simulink model "main_sim_noadapt"  (Simulink 7.2)
settings: Solver=ode2  SolverMode=SingleTasking  StartTime=0.0  StopTime=tsim_max  FixedStep=dtsim  RelTol=1e-3
StopFcn:
  | %mkplt
values from neighbouring files (symbols this model uses):
  vel = 128    [do_command_tracking.m]
undefined symbols (not defined in the file or in its folder): accel_cmd, aero_surf_qbar_off, aero_surf_qbar_on, assertion_time, att_cmd_select, att_trim_IC, att_type, att_type_numbers, bb_ellipsoid, bb_params, chi_trim_IC, command_time, compute_all_rate_cols, compute_all_vel_cols, constants, cosA, da_trim_IC, dc_L2W_IC, de_trim_IC, DiscIntNeverNeededParam, dr_trim_IC, dtsim, E_rwy, E_trim_IC, Ed_cmd, Ed_trim_IC, eow_boundary, flag_exsig, full_surf_llim, full_surf_ulim, gain_set, gain_var_struct, gam_cmd_descent, gam_cmd_preflare, gamdot_cmd_descent, gamdot_cmd_flare, gamdot_cmd_preflare, gamma_trim_IC, h_trim_IC, hd_cmd, hd_trim_IC, ideal_vel_Kb, in_exsig_vecin, in_exsig_vecout, in_t_exsig, MACH, MACH_att_fb, MACH_att_int_IC, MACH_att_Kb, MACH_att_Kc, MACH_att_Ki, MACH_gain_mat, MACH_mass_IC, MACH_pos_IC, MACH_pos_int_IC, MACH_pos_Kb, MACH_pos_Kc, MACH_pos_Ki, MACH_pqr_Bmat_IC, MACH_pqr_IC ... (+62)
libraries: simulink x36, utility_lib x34, mach_lib x24, model_lib x13, simulink_need_slupdate x8, models x8
(part 2 of 7)

== system main_sim_noadapt/vehicle_model/target/seeker model ==
  output_bus : Inport  OutDataType=sfix(16)  OutScaling=2^0
  Bus Selector : BusSelector  OutputSignals=x,xdot
  Bus Selector1 : BusSelector  OutputSignals=LOS_rate,aux_info.azimuth,aux_info.elevation,aux_info.Rground,aux_info.Rslant
  Constant2 : Constant  Value=target_vel_IC  OutDataType=sfix(16)  OutScaling=2^0
  NEh : Selector  InputPortWidth=MACH.num_x  IndexOptions=Index vector (dialog)  Indices=MACH.NEh_idx  OutputSizes=1
  NEh_dot : Selector  InputPortWidth=MACH.num_x  IndexOptions=Index vector (dialog)  Indices=MACH.NEh_idx  OutputSizes=1
  seeker model : Subsystem
  seeker scope : Scope  NumInputPorts=5
      settings: YMin=-1.75~-3.5~-1.75~0~0  YMax=0.25~0.5~0~450000~550000
  target position integrator : Integrator  InitialCondition=target_pos_IC
  seeker : Outport  OutDataType=sfix(16)  OutScaling=2^0
  wires:
  Constant2/1 -> target position integrator/1, seeker model/2(NEh_d_target)
  target position integrator/1 -> seeker model/1(NEh_target)
  NEh/1 -> seeker model/3(NEh)
  NEh_dot/1 -> seeker model/4(NEh_d)
  seeker model/1(seeker) -> seeker/1, Bus Selector1/1
  output_bus/1 -> Bus Selector/1
  Bus Selector/1 -> NEh/1  "<x>"
  Bus Selector/2 -> NEh_dot/1  "<xdot>"
  Bus Selector1/2 -> seeker scope/2  "<azimuth>"
  Bus Selector1/3 -> seeker scope/3  "<elevation>"
  Bus Selector1/4 -> seeker scope/4  "<Rground>"
  Bus Selector1/5 -> seeker scope/5  "<Rslant>"
  Bus Selector1/1 -> seeker scope/1  "<LOS_rate>"

== system main_sim_noadapt/claw_main/att_loops/P+I+AW+TRIM Control ==
  cv : Inport  OutDataType=sfix(16)  OutScaling=2^0
  cv cmd : Inport  Port=2  OutDataType=sfix(16)  OutScaling=2^0
  cvd ff : Inport  Port=3  OutDataType=sfix(16)  OutScaling=2^0
  cvdot extra : Inport  Port=4  OutDataType=sfix(16)  OutScaling=2^0
  trim : Inport  Port=5  OutDataType=sfix(16)  OutScaling=2^0
  reset : Inport  Port=6  OutDataType=sfix(16)  OutScaling=2^0
  x0 : Inport  Port=7  OutDataType=sfix(16)  OutScaling=2^0
  Dot Product2 : simulink/Math Operations/Dot Product  InputSameDT=on  OutDataType=sfix(16)  OutScaling=2^-10  DoSatur=off
  P+I+AW+TRIM Control : mach_lib/P+I+AW+TRIM Control  SystemSampleTime=-1
  Product2 : Product  OutDataType=sfix(16)  OutScaling=2^0  SaturateOnIntegerOverflow=on  InputSameDT=on  OutDataTypeStr=Inherit: Same as first input
  Sum : Sum  Inputs=-+|  OutDataType=sfix(16)  OutScaling=2^0  SaturateOnIntegerOverflow=on
  Unit Delay1 : UnitDelay  SampleTime=-1
  fe : Gain  Gain=MACH.att_fe  ParameterDataType=sfix(16)  ParameterScaling=2^0  OutDataType=sfix(16)  OutScaling=2^0  SaturateOnIntegerOverflow=on  OutDataTypeStr=Inherit: Same as input  ParamDataTypeStr=Inherit: Same as input
  cvdot des : Outport  OutDataType=sfix(16)  OutScaling=2^0
  int state : Outport  Port=2  OutDataType=sfix(16)  OutScaling=2^0
  wires:
  cvd ff/1 -> P+I+AW+TRIM Control/3
  cvdot extra/1 -> P+I+AW+TRIM Control/4
  Sum/1 -> P+I+AW+TRIM Control/5
  reset/1 -> P+I+AW+TRIM Control/6
  x0/1 -> P+I+AW+TRIM Control/7
  fe/1 -> Sum/1
  trim/1 -> Sum/2
  Product2/1 -> fe/1
  Unit Delay1/1 -> Dot Product2/2
  Dot Product2/1 -> Product2/2
  P+I+AW+TRIM Control/2 -> int state/1
  P+I+AW+TRIM Control/1 -> Unit Delay1/1, cvdot des/1
  cv cmd/1 -> P+I+AW+TRIM Control/2
  cv/1 -> Product2/1, Dot Product2/1, P+I+AW+TRIM Control/1

== system main_sim_noadapt/claw_main/att_loops/compute trim ==
  inner cmd : Inport  OutDataType=sfix(16)  OutScaling=2^0
  Bmat : Inport  Port=2  OutDataType=sfix(16)  OutScaling=2^0
  cmd : Inport  Port=3  OutDataType=sfix(16)  OutScaling=2^0
  Product : Product  Multiplication=Matrix(*)  OutDataType=sfix(16)  OutScaling=2^0  SaturateOnIntegerOverflow=on  OutDataTypeStr=Inherit: Same as first input
  Sum1 : Sum  Inputs=|+-  OutDataType=sfix(16)  OutScaling=2^0  SaturateOnIntegerOverflow=on
  trim : Outport  OutDataType=sfix(16)  OutScaling=2^0
  wires:
  Product/1 -> trim/1
  Bmat/1 -> Product/1
  Sum1/1 -> Product/2
  inner cmd/1 -> Sum1/1
  cmd/1 -> Sum1/2

== system main_sim_noadapt/claw_main/att_loops/dyn inv ==
  limit_pqr_cmd : Inport  OutDataType=sfix(16)  OutScaling=2^0
  uvw : Inport  Port=2  OutDataType=sfix(16)  OutScaling=2^0
  e nom : Inport  Port=3  OutDataType=sfix(16)  OutScaling=2^0
  e dot des : Inport  Port=4  OutDataType=sfix(16)  OutScaling=2^0
  Dot Product : simulink/Math Operations/Dot Product  InputSameDT=on  OutDataType=sfix(16)  OutScaling=2^-10  DoSatur=off
  Gain4 : Gain  Gain=0.5  ParameterDataType=sfix(16)  ParameterScaling=2^0  OutDataType=sfix(16)  OutScaling=2^0
  Limit rate cmd : Subsystem
  Product4 : Product  OutDataType=sfix(16)  OutScaling=2^0  SaturateOnIntegerOverflow=on  InputSameDT=on  OutDataTypeStr=Inherit: Same as first input
  Product5 : Product  Inputs=**  Multiplication=Matrix(*)  OutDataType=sfix(16)  OutScaling=2^0  SaturateOnIntegerOverflow=on  InputSameDT=on  OutDataTypeStr=Inherit: Same as first input
  Sum4 : Sum  Inputs=++-  OutDataType=sfix(16)  OutScaling=2^0  SaturateOnIntegerOverflow=on  InputSameDT=on  OutDataTypeStr=Inherit: Same as first input
  getedinv : utility_lib/getedinv  SystemSampleTime=-1
  Bmat : Outport  OutDataType=sfix(16)  OutScaling=2^0
  pqr : Outport  Port=2  OutDataType=sfix(16)  OutScaling=2^0
  cvdex : Outport  Port=3  OutDataType=sfix(16)  OutScaling=2^0
  wires:
  Limit rate cmd/1(pqr_limited) -> pqr/1, Product5/2
  Sum4/1 -> cvdex/1
  Product4/1 -> Sum4/2
  Product5/1 -> Sum4/1
  e dot des/1 -> Dot Product/2, Sum4/3, getedinv/1
  e nom/1 -> Product4/1, Dot Product/1, getedinv/2
  Dot Product/1 -> Product4/2
  getedinv/2 -> Gain4/1
  uvw/1 -> Limit rate cmd/2(uvw)
  getedinv/1 -> Limit rate cmd/3(pqr)
  limit_pqr_cmd/1 -> Limit rate cmd/1(limit_pqr_cmd)
  Gain4/1 -> Product5/1, Bmat/1

== system main_sim_noadapt/claw_main/att_loops/low pass filter ==
  e_cmd : Inport  OutDataType=sfix(16)  OutScaling=2^0
  signal_bus : Inport  Port=2  OutDataType=sfix(16)  OutScaling=2^0
  att_ff : Inport  Port=3  OutDataType=sfix(16)  OutScaling=2^0
  Bus Selector4 : BusSelector  OutputSignals=control_params.att_desdyn.kf,control_params.att_desdyn.kb
  Compare To Zero : simulink/Logic and Bit Operations/Compare To Zero  SystemSampleTime=-1  relop===  LogicOutDataTypeMode=boolean  ZeroCross=off
  Constant : Constant  Value=MACH_att_fb  OutDataType=sfix(16)  OutScaling=2^0
  Discrete-Time Integrator : DiscreteIntegrator  ExternalReset=sampled level  InitialConditionSource=external  SampleTime=-1  OutDataType=sfix(16)  OutScaling=2^0  ICPrevOutput=DiscIntNeverNeededParam  ICPrevScaledInput=DiscIntNeverNeededParam
  Product : Product  Inputs=3  OutDataType=sfix(16)  OutScaling=2^0  RndMeth=Zero
  Product1 : Product  OutDataType=sfix(16)  OutScaling=2^0  RndMeth=Zero
  Product2 : Product  OutDataType=sfix(16)  OutScaling=2^0  RndMeth=Zero
  Sum : Sum  Inputs=|+-  OutDataType=sfix(16)  OutScaling=2^0
  Sum1 : Sum  Inputs=++|  OutDataType=sfix(16)  OutScaling=2^0
  cv cmd : Outport  OutDataType=sfix(16)  OutScaling=2^0
  cvd ff : Outport  Port=2  OutDataType=sfix(16)  OutScaling=2^0
  wires:
  Product/1 -> Sum1/2
  e_cmd/1 -> Sum/1, Discrete-Time Integrator/3
  Sum/1 -> Product/3
  Sum1/1 -> Discrete-Time Integrator/1, cvd ff/1
  Discrete-Time Integrator/1 -> Sum/2, cv cmd/1
  signal_bus/1 -> Bus Selector4/1
  att_ff/1 -> Product1/1
  Product1/1 -> Sum1/1
  Compare To Zero/1 -> Discrete-Time Integrator/2
  Bus Selector4/2 -> Product/2  "<kb>"
  Product2/1 -> Product/1, Compare To Zero/1
  Bus Selector4/1 -> Product2/2, Product1/2  "<kf>"
  Constant/1 -> Product2/1

== system main_sim_noadapt/claw_main/att_loops/select att cmd ==
  e_current : Inport  OutDataType=sfix(16)  OutScaling=2^0
  throt_current : Inport  Port=2  OutDataType=sfix(16)  OutScaling=2^0
  outer cmd : Inport  Port=3  OutDataType=sfix(16)  OutScaling=2^0
  signal_bus : Inport  Port=4  OutDataType=sfix(16)  OutScaling=2^0
  Bus Selector1 : BusSelector  OutputSignals=cmd_bus.select_cmd.att
  Compare To Zero : simulink/Logic and Bit Operations/Compare To Zero  SystemSampleTime=-1  relop===  LogicOutDataTypeMode=boolean  ZeroCross=off
  Demux : Demux  Outputs=[ 4 1 ]
  Demux1 : Demux  Outputs=[ 3 MACH.num_u_throt ]
  Demux2 : Demux  Outputs=[ 1 3 ]
  Mux1 : Mux  Inputs=2
  Switch : Switch  Threshold=0.5
  Unit Delay2 : UnitDelay  X0=MACH_throttle_IC  SampleTime=-1
  att2e_ref : utility_lib/att2e_ref  SystemSampleTime=-1
  e2att : utility_lib/e2att  SystemSampleTime=-1
  get direct cmd : Subsystem
  switch att cmd : MultiPortSwitch  zeroidx=on  SaturateOnIntegerOverflow=on
  switch throt cmd : MultiPortSwitch  zeroidx=on  SaturateOnIntegerOverflow=on
  e_cmd : Outport  OutDataType=sfix(16)  OutScaling=2^0
  throt_cmd : Outport  Port=2  OutDataType=sfix(16)  OutScaling=2^0
  cmd : Outport  Port=3  OutDataType=sfix(16)  OutScaling=2^0
  wires:
  switch att cmd/1 -> att2e_ref/1, Mux1/1
  Bus Selector1/1 -> Demux/1  "<att>"
  get direct cmd/2(throt) -> switch throt cmd/3
  throt_current/1 -> Unit Delay2/1
  Demux/2 -> switch throt cmd/1
  outer cmd/1 -> Demux1/1
  Demux1/2 -> switch throt cmd/4
  switch throt cmd/1 -> throt_cmd/1, Mux1/2
  signal_bus/1 -> get direct cmd/1(signal_bus), Bus Selector1/1
  Demux/1 -> Demux2/1
  e_current/1 -> e2att/1, Switch/1, att2e_ref/2
  Unit Delay2/1 -> switch throt cmd/2
  get direct cmd/1(att) -> switch att cmd/3
  e2att/1 -> switch att cmd/2
  Demux1/1 -> switch att cmd/4
  att2e_ref/1 -> Switch/3
  Switch/1 -> e_cmd/1
  Demux2/1 -> Compare To Zero/1
  Demux2/2 -> switch att cmd/1
  Compare To Zero/1 -> Switch/2
  Mux1/1 -> cmd/1

== system main_sim_noadapt/claw_main/grab ExportedGlobal/grab cv variables ==
  In1 : Inport  OutDataType=sfix(16)  OutScaling=2^0
  Bus Selector6 : BusSelector  OutputSignals=rate.cv,att.cv,vel.cv,pos.cv
  Demux1 : Demux  Outputs=3
  Demux2 : Demux
  Demux3 : Demux  Outputs=3
  Demux4 : Demux  Outputs=3
  Mux : Mux  Inputs=13
  Subsystem : Subsystem  TreatAsAtomicUnit=on
      settings: RTWSystemCode=Inline
  Out1 : Outport  OutDataType=sfix(16)  OutScaling=2^0
  wires:
  Subsystem/1(Out1) -> Mux/1  "CLAW_p_cv"
  Subsystem/2(Out2) -> Mux/2  "CLAW_q_cv"
  Subsystem/3(Out3) -> Mux/3  "CLAW_r_cv"
  Subsystem/4(Out4) -> Mux/4  "CLAW_e0_cv"
  Subsystem/5(Out5) -> Mux/5  "CLAW_e1_cv"
  Subsystem/6(Out6) -> Mux/6  "CLAW_e2_cv"
  Subsystem/8(Out8) -> Mux/8  "CLAW_Ndot_cv"
  Subsystem/9(Out9) -> Mux/9  "CLAW_Edot_cv"
  Subsystem/10(Out10) -> Mux/10  "CLAW_hdot_cv"
  Subsystem/11(Out11) -> Mux/11  "CLAW_N_cv"
  Subsystem/12(Out12) -> Mux/12  "CLAW_E_cv"
  Subsystem/13(Out13) -> Mux/13  "CLAW_h_cv"
  Subsystem/7(Out7) -> Mux/7  "CLAW_e3_cv"
  In1/1 -> Bus Selector6/1
  Mux/1 -> Out1/1
  Demux1/1 -> Subsystem/1(In1)
  Demux1/2 -> Subsystem/2(In2)
  Demux1/3 -> Subsystem/3(In3)
  Demux2/1 -> Subsystem/4(In4)
  Demux2/2 -> Subsystem/5(In5)
  Demux2/3 -> Subsystem/6(In6)
  Demux2/4 -> Subsystem/7(In7)
  Demux3/1 -> Subsystem/8(In8)
  Demux3/2 -> Subsystem/9(In9)
  Demux3/3 -> Subsystem/10(In10)
  Demux4/1 -> Subsystem/11(In11)
  Demux4/2 -> Subsystem/12(In12)
  Demux4/3 -> Subsystem/13(In13)
  Bus Selector6/1 -> Demux1/1  "<cv>"
  Bus Selector6/2 -> Demux2/1  "<cv>"
  Bus Selector6/3 -> Demux3/1  "<cv>"
  Bus Selector6/4 -> Demux4/1  "<cv>"

== system main_sim_noadapt/claw_main/grab ExportedGlobal/grab cvcmd variables ==
  In1 : Inport  OutDataType=sfix(16)  OutScaling=2^0
  Bus Selector5 : BusSelector  OutputSignals=rate.cvc,att.cvc,vel.cvc,pos.cvc
  Demux1 : Demux  Outputs=3
  Demux2 : Demux
  Demux3 : Demux  Outputs=3
  Demux4 : Demux  Outputs=3
  Mux : Mux  Inputs=13
  Subsystem : Subsystem  TreatAsAtomicUnit=on
      settings: RTWSystemCode=Inline
  Out1 : Outport  OutDataType=sfix(16)  OutScaling=2^0
  wires:
  Subsystem/1(Out1) -> Mux/1  "CLAW_p_cvcmd"
  Subsystem/2(Out2) -> Mux/2  "CLAW_q_cvcmd"
  Subsystem/3(Out3) -> Mux/3  "CLAW_r_cvcmd"
  Subsystem/4(Out4) -> Mux/4  "CLAW_e0_cvcmd"
  Subsystem/5(Out5) -> Mux/5  "CLAW_e1_cvcmd"
  Subsystem/6(Out6) -> Mux/6  "CLAW_e2_cvcmd"
  Subsystem/8(Out8) -> Mux/8  "CLAW_Ndot_cvcmd"
  Subsystem/9(Out9) -> Mux/9  "CLAW_Edot_cvcmd"
  Subsystem/10(Out10) -> Mux/10  "CLAW_hdot_cvcmd"
  Subsystem/11(Out11) -> Mux/11  "CLAW_N_cvcmd"
  Subsystem/12(Out12) -> Mux/12  "CLAW_E_cvcmd"
  Subsystem/13(Out13) -> Mux/13  "CLAW_h_cvcmd"
  Subsystem/7(Out7) -> Mux/7  "CLAW_e3_cvcmd"
  In1/1 -> Bus Selector5/1
  Mux/1 -> Out1/1
  Demux1/1 -> Subsystem/1(In1)
  Demux1/2 -> Subsystem/2(In2)
  Demux1/3 -> Subsystem/3(In3)
  Demux2/1 -> Subsystem/4(In4)
  Demux2/2 -> Subsystem/5(In5)
  Demux2/3 -> Subsystem/6(In6)
  Demux2/4 -> Subsystem/7(In7)
  Demux3/1 -> Subsystem/8(In8)
  Demux3/2 -> Subsystem/9(In9)
  Demux3/3 -> Subsystem/10(In10)
  Demux4/1 -> Subsystem/11(In11)
  Demux4/2 -> Subsystem/12(In12)
  Demux4/3 -> Subsystem/13(In13)
  Bus Selector5/4 -> Demux4/1  "<cvc>"
  Bus Selector5/2 -> Demux2/1  "<cvc>"
  Bus Selector5/1 -> Demux1/1  "<cvc>"
  Bus Selector5/3 -> Demux3/1  "<cvc>"

== system main_sim_noadapt/claw_main/grab ExportedGlobal/grab cvdex variables ==
  In1 : Inport  OutDataType=sfix(16)  OutScaling=2^0
  Bus Selector3 : BusSelector  OutputSignals=rate.cvdex,att.cvdex,vel.cvdex,pos.cvdex
  Demux1 : Demux  Outputs=3
  Demux2 : Demux
  Demux3 : Demux  Outputs=3
  Demux4 : Demux  Outputs=3
  Mux : Mux  Inputs=13
  Subsystem : Subsystem  TreatAsAtomicUnit=on
      settings: RTWSystemCode=Inline
  Out1 : Outport  OutDataType=sfix(16)  OutScaling=2^0
  wires:
  Subsystem/1(Out1) -> Mux/1  "CLAW_p_cvdex"
  Subsystem/2(Out2) -> Mux/2  "CLAW_q_cvdex"
  Subsystem/3(Out3) -> Mux/3  "CLAW_r_cvdex"
  Subsystem/4(Out4) -> Mux/4  "CLAW_e0_cvdex"
  Subsystem/5(Out5) -> Mux/5  "CLAW_e1_cvdex"
  Subsystem/6(Out6) -> Mux/6  "CLAW_e2_cvdex"
  Subsystem/8(Out8) -> Mux/8  "CLAW_Ndot_cvdex"
  Subsystem/9(Out9) -> Mux/9  "CLAW_Edot_cvdex"
  Subsystem/10(Out10) -> Mux/10  "CLAW_hdot_cvdex"
  Subsystem/11(Out11) -> Mux/11  "CLAW_N_cvdex"
  Subsystem/12(Out12) -> Mux/12  "CLAW_E_cvdex"
  Subsystem/13(Out13) -> Mux/13  "CLAW_h_cvdex"
  Subsystem/7(Out7) -> Mux/7  "CLAW_e3_cvdex"
  Demux1/1 -> Subsystem/1(In1)
  Demux1/2 -> Subsystem/2(In2)
  Demux1/3 -> Subsystem/3(In3)
  Demux2/1 -> Subsystem/4(In4)
  Demux2/2 -> Subsystem/5(In5)
  Demux2/3 -> Subsystem/6(In6)
  Demux2/4 -> Subsystem/7(In7)
  Demux3/1 -> Subsystem/8(In8)
  Demux3/2 -> Subsystem/9(In9)
  Demux3/3 -> Subsystem/10(In10)
  Demux4/1 -> Subsystem/11(In11)
  Demux4/2 -> Subsystem/12(In12)
  Demux4/3 -> Subsystem/13(In13)
  Mux/1 -> Out1/1
  In1/1 -> Bus Selector3/1
  Bus Selector3/4 -> Demux4/1  "<cvdex>"
  Bus Selector3/3 -> Demux3/1  "<cvdex>"
  Bus Selector3/2 -> Demux2/1  "<cvdex>"
  Bus Selector3/1 -> Demux1/1  "<cvdex>"

== system main_sim_noadapt/claw_main/grab ExportedGlobal/grab integrator variables ==
  In1 : Inport  OutDataType=sfix(16)  OutScaling=2^0
  Bus Selector4 : BusSelector  OutputSignals=rate.integ,att.integ,vel.integ,pos.integ
  Demux1 : Demux  Outputs=3
  Demux2 : Demux
  Demux3 : Demux  Outputs=3
  Demux4 : Demux  Outputs=3
  Mux : Mux  Inputs=13
  Subsystem : Subsystem  TreatAsAtomicUnit=on
      settings: RTWSystemCode=Inline
  Out1 : Outport  OutDataType=sfix(16)  OutScaling=2^0
  wires:
  Subsystem/1(Out1) -> Mux/1  "CLAW_p_int"
  Subsystem/2(Out2) -> Mux/2  "CLAW_q_int"
  Subsystem/3(Out3) -> Mux/3  "CLAW_r_int"
  Subsystem/4(Out4) -> Mux/4  "CLAW_e0_int"
  Subsystem/5(Out5) -> Mux/5  "CLAW_e1_int"
  Subsystem/6(Out6) -> Mux/6  "CLAW_e2_int"
  Subsystem/8(Out8) -> Mux/8  "CLAW_Ndot_int"
  Subsystem/9(Out9) -> Mux/9  "CLAW_Edot_int"
  Subsystem/10(Out10) -> Mux/10  "CLAW_hdot_int"
  Subsystem/11(Out11) -> Mux/11  "CLAW_N_int"
  Subsystem/12(Out12) -> Mux/12  "CLAW_E_int"
  Subsystem/13(Out13) -> Mux/13  "CLAW_h_int"
  Subsystem/7(Out7) -> Mux/7  "CLAW_e3_int"
  Mux/1 -> Out1/1
  Demux1/1 -> Subsystem/1(In1)
  Demux1/2 -> Subsystem/2(In2)
  Demux1/3 -> Subsystem/3(In3)
  Demux2/1 -> Subsystem/4(In4)
  Demux2/2 -> Subsystem/5(In5)
  Demux2/3 -> Subsystem/6(In6)
  Demux2/4 -> Subsystem/7(In7)
  Demux3/1 -> Subsystem/8(In8)
  Demux3/2 -> Subsystem/9(In9)
  Demux3/3 -> Subsystem/10(In10)
  Demux4/1 -> Subsystem/11(In11)
  Demux4/2 -> Subsystem/12(In12)
  Demux4/3 -> Subsystem/13(In13)
  In1/1 -> Bus Selector4/1
  Bus Selector4/4 -> Demux4/1  "<integ>"
  Bus Selector4/3 -> Demux3/1  "<integ>"
  Bus Selector4/2 -> Demux2/1  "<integ>"
  Bus Selector4/1 -> Demux1/1  "<integ>"

== system main_sim_noadapt/claw_main/grab ExportedGlobal/grab w_est variables ==
  In1 : Inport  OutDataType=sfix(16)  OutScaling=2^0
  Bus Selector12 : BusSelector  OutputSignals=w_est_debug.w_est
  Demux1 : Demux  Outputs=3
  Mux : Mux  Inputs=3
  Subsystem : Subsystem  TreatAsAtomicUnit=on
      settings: RTWSystemCode=Inline
  Out1 : Outport  OutDataType=sfix(16)  OutScaling=2^0
  wires:
  Subsystem/1(Out1) -> Mux/1  "CLAW_Nd_wind"
  Subsystem/2(Out2) -> Mux/2  "CLAW_Ed_wind"
  Subsystem/3(Out3) -> Mux/3  "CLAW_Dd_wind"
  Demux1/1 -> Subsystem/1(In1)
  Demux1/2 -> Subsystem/2(In2)
  Demux1/3 -> Subsystem/3(In3)
  Mux/1 -> Out1/1
  Bus Selector12/1 -> Demux1/1  "<w_est>"
  In1/1 -> Bus Selector12/1

== system main_sim_noadapt/claw_main/input processing/mode dependent stick processing ==
  command : Inport  OutDataType=sfix(16)  OutScaling=2^0
  signal_bus : Inport  Port=2  OutDataType=sfix(16)  OutScaling=2^0
  Bus Creator : BusCreator  Inputs=2
  Bus Selector1 : BusSelector  OutputSignals=control_params.accel_cmd_sw,mode_sw.CLAW_mode
  Bus Selector2 : BusSelector  OutputSignals=y_meas.NEh_dot,x_est
  att rate cmd : Subsystem
  att_type cmd : Subsystem
  feed forward : Subsystem
  llh cmd : Subsystem
  rampin vel_cmd : Subsystem
  set command selection switches : Subsystem
  table iv computation : Subsystem
  use table lookup pos cmds : Subsystem
  cmd_bus : Outport  OutDataType=sfix(16)  OutScaling=2^0
  feed_forward : Outport  Port=2  OutDataType=sfix(16)  OutScaling=2^0
  wires:
  Bus Selector1/2 -> set command selection switches/2(CLAW_mode), att rate cmd/1(mode), llh cmd/1(mode), rampin vel_cmd/1(mode), use table lookup pos cmds/1(mode), att_type cmd/1(mode)  "<CLAW_mode>"
  signal_bus/1 -> Bus Selector1/1, llh cmd/3(signal_bus), att rate cmd/3(signal_bus), Bus Selector2/1, att_type cmd/3(signal_bus), feed forward/2(signal_bus)
  llh cmd/1(command_out) -> att rate cmd/2(command_in)
  Bus Selector2/1 -> rampin vel_cmd/3(NEh_dot)  "<NEh_dot>"
  Bus Selector1/1 -> set command selection switches/1(accel_cmd_sw)  "<accel_cmd_sw>"
  set command selection switches/1(select_cmd) -> Bus Creator/1  "select_cmd"
  rampin vel_cmd/1(command_out) -> use table lookup pos cmds/2(command_in)
  Bus Creator/1 -> cmd_bus/1
  use table lookup pos cmds/1(command_out) -> Bus Creator/2  "autopilot_cmd"
  Bus Selector2/2 -> table iv computation/1(x_est)  "<x_est>"
  table iv computation/1(table_bus) -> use table lookup pos cmds/3(table_bus), feed forward/1(table_bus)
  feed forward/1(feed_forward) -> feed_forward/1
  command/1 -> llh cmd/2(command_in)
  att_type cmd/1(command_out) -> rampin vel_cmd/2(command_in)
  att rate cmd/1(command_out) -> att_type cmd/2(command_in)

== system main_sim_noadapt/claw_main/input processing/modify limits and apply to direct commands ==
  note: Currently, the limits for direct mode and throttle in att and rate modes
      | are the same as those used for automatic control.  May want to revisit this someday ...
  u_old : Inport  OutDataType=sfix(16)  OutScaling=2^0
  u_meas : Inport  Port=2  OutDataType=sfix(16)  OutScaling=2^0
  full_surf_in : Inport  Port=3  OutDataType=sfix(16)  OutScaling=2^0
  Bus Assignment : BusAssignment  AssignedSignals=full_surf_cmd
  Bus Selector2 : BusSelector  OutputSignals=full_surf_ulim,full_surf_llim,full_surf_urlim,full_surf_lrlim,full_surf_cmd
  MinMax : MinMax  Inputs=2  OutDataType=sfix(16)  OutScaling=2^0  SaturateOnIntegerOverflow=on  InputSameDT=on
  MinMax2 : MinMax  Function=max  Inputs=2  OutDataType=sfix(16)  OutScaling=2^0  SaturateOnIntegerOverflow=on  InputSameDT=on
  apply surface locking : Subsystem
  limit computation : mach_lib/limit computation  SystemSampleTime=-1
  rate limit limits : mach_lib/rate limit limits  SystemSampleTime=-1  ulim=MACH.u_ulim  llim=MACH.u_llim
  throt out of fuel limits : Subsystem
  full_surf : Outport  OutDataType=sfix(16)  OutScaling=2^0
  wires:
  Bus Selector2/3 -> rate limit limits/4, limit computation/4  "<full_surf_urlim>"
  Bus Selector2/4 -> rate limit limits/5, limit computation/5  "<full_surf_lrlim>"
  rate limit limits/1 -> limit computation/2
  rate limit limits/2 -> limit computation/3
  limit computation/2 -> MinMax2/1
  limit computation/1 -> MinMax/1
  MinMax2/1 -> MinMax/2
  u_old/1 -> rate limit limits/1, limit computation/1
  Bus Selector2/2 -> rate limit limits/3  "<full_surf_llim>"
  Bus Selector2/5 -> MinMax2/2  "<full_surf_cmd>"
  MinMax/1 -> Bus Assignment/2
  throt out of fuel limits/1(full_surf) -> Bus Selector2/1, Bus Assignment/1
  Bus Selector2/1 -> rate limit limits/2  "<full_surf_ulim>"
  Bus Assignment/1 -> full_surf/1
  u_meas/1 -> apply surface locking/1(u_meas)
  full_surf_in/1 -> apply surface locking/2(full_surf_in)
  apply surface locking/1(full_surf) -> throt out of fuel limits/1(full_surf_in)

== system main_sim_noadapt/claw_main/input processing/select att_type ==
  scoped_bus : Inport  OutDataType=sfix(16)  OutScaling=2^0
  mode_sw_in : Inport  Port=2  OutDataType=sfix(16)  OutScaling=2^0
  signal_bus : Inport  Port=3  OutDataType=sfix(16)  OutScaling=2^0
  Bus Assignment : BusAssignment  AssignedSignals=att_type
  Bus Selector : BusSelector  OutputSignals=qbar,abs_vel_rw,abs_cos_beta,abs_cos_theta,abs_cos_b,abs_cos_gamma_rw
  Bus Selector1 : BusSelector  OutputSignals=att_type
  Constant5 : Constant  Value=use_auto_att_type  OutDataType=sfix(16)  OutScaling=2^0
  Multiport Switch1 : MultiPortSwitch  Inputs=2  zeroidx=on
  Product : Product  OutDataType=sfix(16)  OutScaling=2^0  RndMeth=Zero
  add tiebreaker for current att_type : Subsystem
  att type input : Scope  NumInputPorts=6
      settings: YMin=1~0~0~0.1~5.55112e-017~5.55112e-017  YMax=4~900~5000~1~1~1  SaveName=att_type_input
  att type output : Scope  NumInputPorts=2
      settings: YMin=1~0  YMax=4~2.5  SaveName=att_type_output
  compute precond vars : Subsystem
  evaluate preconditions : Subsystem
  priority_weighting : Constant  Value=[0 1 1 0 2 0]  OutDataType=sfix(16)  OutScaling=2^0
  select best att_type : Subsystem
  mode_sw : Outport  OutDataType=sfix(16)  OutScaling=2^0
  wires:
  scoped_bus/1 -> compute precond vars/2(scoped_bus)
  mode_sw_in/1 -> Bus Selector1/1, Bus Assignment/1
  signal_bus/1 -> compute precond vars/1(signal_bus)
  Bus Selector1/1 -> Multiport Switch1/2  "<att_type>"
  Bus Assignment/1 -> mode_sw/1
  add tiebreaker for current att_type/1(priority_out) -> Product/1
  Product/1 -> select best att_type/1(vec), att type output/2  "att_type_availability"
  select best att_type/1(idx_max) -> att type output/1, Multiport Switch1/3, add tiebreaker for current att_type/1(att_type_selected)  "att_type_selected"
  evaluate preconditions/1(precond_satisfied) -> Product/2
  Multiport Switch1/1 -> Bus Assignment/2
  Constant5/1 -> Multiport Switch1/1
  priority_weighting/1 -> add tiebreaker for current att_type/2(priority_in)
  compute precond vars/1(precond_vars) -> Bus Selector/1, evaluate preconditions/1(precond_vars)
  Bus Selector/1 -> att type input/1  "<qbar>"
  Bus Selector/2 -> att type input/2  "<abs_vel_rw>"
  Bus Selector/3 -> att type input/3  "<abs_cos_beta>"
  Bus Selector/4 -> att type input/4  "<abs_cos_theta>"
  Bus Selector/5 -> att type input/5  "<abs_cos_b>"
  Bus Selector/6 -> att type input/6  "<abs_cos_gamma_rw>"

== system main_sim_noadapt/claw_main/input processing/set control parameters ==
  note: (Optionally) disable bb
      |  while we still have fuel
  signal_bus : Inport  OutDataType=sfix(16)  OutScaling=2^0
  full_surf : Inport  Port=2  OutDataType=sfix(16)  OutScaling=2^0
  Bus Creator1 : BusCreator  Inputs=10
  Bus Selector1 : BusSelector  OutputSignals=mode_sw.enable_bb_sw,mode_sw.gain_set_sw
  Bus Selector3 : BusSelector  OutputSignals=aero_env_est
  Constant : Constant  OutDataType=sfix(16)  OutScaling=2^0
  Constant1 : Constant  OutDataType=sfix(16)  OutScaling=2^0
  Logical Operator : Logic  Operator=NOT  AllPortsSameDT=off
  Logical Operator1 : Logic  Operator=NOT  AllPortsSameDT=off
  Logical Operator4 : Logic  AllPortsSameDT=off
  Logical Operator5 : Logic  Operator=OR  AllPortsSameDT=off
  accel submode setup : Subsystem
  modify MACH_att_Kf : Subsystem
  out of fuel : model_lib/out of fuel ?  SystemSampleTime=-1
  select gains : Subsystem
  set att desdyn params : Subsystem
  set pos desdyn params : Subsystem
  set rate desdyn params : Subsystem
  set rate di params : Subsystem
  set vel desdyn params : Subsystem
  control_params : Outport  OutDataType=sfix(16)  OutScaling=2^0
  wires:
  set pos desdyn params/1(params) -> Bus Creator1/6  "pos_desdyn"
  set vel desdyn params/1(params) -> Bus Creator1/7  "vel_desdyn"
  set att desdyn params/1(params) -> Bus Creator1/8  "att_desdyn"
  set rate desdyn params/1(params) -> Bus Creator1/9  "rate_desdyn"
  Bus Selector1/1 -> Logical Operator4/1  "<enable_bb_sw>"
  Logical Operator/1 -> Bus Creator1/3  "limit_pqr_cmd"
  Logical Operator4/1 -> select gains/1(enable_bb), Logical Operator/1, Bus Creator1/4  "enable_bb"
  select gains/2(gain_bus) -> set pos desdyn params/1(gain_bus), set vel desdyn params/1(gain_bus), set rate desdyn params/1(gain_bus), modify MACH_att_Kf/1(gain_bus_in)
  Bus Creator1/1 -> control_params/1
  select gains/1(gain_set) -> Bus Creator1/5  "gain_set"
  Constant/1 -> out of fuel/1
  out of fuel/1 -> Logical Operator1/1
  Logical Operator1/1 -> Logical Operator5/1
  Logical Operator5/1 -> Logical Operator4/2
  Constant1/1 -> Logical Operator5/2
  Bus Selector1/2 -> select gains/2(gain_set_in)  "<gain_set_sw>"
  accel submode setup/2(accel_cmd) -> Bus Creator1/2  "accel_cmd"
  accel submode setup/1(accel_cmd_sw) -> Bus Creator1/1  "accel_cmd_sw"
  signal_bus/1 -> accel submode setup/1(signal_bus), Bus Selector1/1, Bus Selector3/1, modify MACH_att_Kf/2(signal_bus)
  set rate di params/1(rate_params) -> Bus Creator1/10  "rate_params"
  Bus Selector3/1 -> set rate di params/2(aero_env_est)  "<aero_env_est>"
  full_surf/1 -> set rate di params/1(full_surf)
  modify MACH_att_Kf/1(gain_bus) -> set att desdyn params/1(gain_bus)

== system main_sim_noadapt/claw_main/pos_loops/compute trim ==
  inner cmd : Inport  OutDataType=sfix(16)  OutScaling=2^0
  cmd : Inport  Port=2  OutDataType=sfix(16)  OutScaling=2^0
  Sum1 : Sum  Inputs=|+-  OutDataType=sfix(16)  OutScaling=2^0  SaturateOnIntegerOverflow=on
  trim : Outport  OutDataType=sfix(16)  OutScaling=2^0
  wires:
  Sum1/1 -> trim/1
  inner cmd/1 -> Sum1/1
  cmd/1 -> Sum1/2

== system main_sim_noadapt/claw_main/pos_loops/limiter ==
  vel_inner_cmd : Inport  OutDataType=sfix(16)  OutScaling=2^0
  signal_bus : Inport  Port=2  OutDataType=sfix(16)  OutScaling=2^0
  cvd_des_in : Inport  Port=3  OutDataType=sfix(16)  OutScaling=2^0
  Bus Selector2 : BusSelector  OutputSignals=cmd_bus.select_cmd.vel,feed_forward.pos_ff,y_meas.dc_fltpath
  Compare To Constant : simulink/Logic and Bit Operations/Compare To Constant  SystemSampleTime=-1  relop=<  const=2  LogicOutDataTypeMode=boolean  ZeroCross=off
  Constant : Constant  Value=use_pos_fltpath_lim  OutDataType=sfix(16)  OutScaling=2^0
  Math Function : Math  Operator=transpose  OutDataType=sfix(16)  OutScaling=2^0  SaturateOnIntegerOverflow=on
  Product : Product  Multiplication=Matrix(*)  OutDataType=sfix(16)  OutScaling=2^0  RndMeth=Zero
  Product1 : Product  Multiplication=Matrix(*)  OutDataType=sfix(16)  OutScaling=2^0  RndMeth=Zero
  Saturation : Saturate  UpperLimit=MACH.pos_u_ulim  LowerLimit=MACH.pos_u_llim
  Saturation1 : Saturate  UpperLimit=MACH.pos_fltpath_u_ulim  LowerLimit=MACH.pos_fltpath_u_llim
  Selector1 : Selector  InputPortWidth=4  IndexOptions=Index vector (dialog)  Indices=[1 2 4]  OutputSizes=1
  Sum : Sum  Inputs=-+|  OutDataType=sfix(16)  OutScaling=2^0
  Sum1 : Sum  Inputs=++|  OutDataType=sfix(16)  OutScaling=2^0
  Sum2 : Sum  Inputs=+-|  OutDataType=sfix(16)  OutScaling=2^0  SaturateOnIntegerOverflow=on  InputSameDT=on  OutDataTypeStr=Inherit: Same as first input
  Switch : Switch  Threshold=0.5
  Switch1 : Switch  Threshold=0.5
  Unit Delay : UnitDelay  X0=MACH_vel_IC  SampleTime=MACH.dt
  cvd_des : Outport  OutDataType=sfix(16)  OutScaling=2^0
  cvd_extra : Outport  Port=2  OutDataType=sfix(16)  OutScaling=2^0
  wires:
  Switch1/1 -> Sum1/1, Sum/1
  Constant/1 -> Switch/2
  Saturation/1 -> Switch/3
  Switch/1 -> cvd_des/1, Sum2/1
  Sum1/1 -> Switch/1
  cvd_des_in/1 -> Sum/2, Saturation/1, Sum2/2
  Bus Selector2/3 -> Product/1, Math Function/1  "<dc_fltpath>"
  Sum/1 -> Product/2
  Product/1 -> Saturation1/1
  Saturation1/1 -> Product1/2
  Math Function/1 -> Product1/1
  Product1/1 -> Sum1/2
  Sum2/1 -> cvd_extra/1
  signal_bus/1 -> Bus Selector2/1
  Bus Selector2/1 -> Selector1/1  "<vel>"
  Bus Selector2/2 -> Switch1/3  "<pos_ff>"
  Compare To Constant/1 -> Switch1/2
  Selector1/1 -> Compare To Constant/1
  Unit Delay/1 -> Switch1/1
  vel_inner_cmd/1 -> Unit Delay/1

== system main_sim_noadapt/claw_main/pos_loops/select pos cmd ==
  NEh_current : Inport  OutDataType=sfix(16)  OutScaling=2^0
  outer cmd : Inport  Port=2  OutDataType=sfix(16)  OutScaling=2^0
  signal_bus : Inport  Port=3  OutDataType=sfix(16)  OutScaling=2^0
  Bus Selector : BusSelector  OutputSignals=cmd_bus.select_cmd.pos,cmd_bus.autopilot_cmd
  Demux3 : Demux  Outputs=[ 3 1 ]
  Ground : Ground
  Multiport Switch : MultiPortSwitch  zeroidx=on  SaturateOnIntegerOverflow=on
  Mux1 : Mux  Inputs=2
  Selector2 : Selector  InputPortWidth=4  IndexOptions=Index vector (dialog)  Indices=[1 2 4 3]  OutputSizes=1
  Selector4 : Selector  InputPortWidth=4  IndexOptions=Index vector (dialog)  Indices=[1 2 4 3]  OutputSizes=1
  NEh_cmd : Outport  OutDataType=sfix(16)  OutScaling=2^0
  cam_cmd : Outport  Port=2  OutDataType=sfix(16)  OutScaling=2^0
  cmd : Outport  Port=3  OutDataType=sfix(16)  OutScaling=2^0
  wires:
  Multiport Switch/1 -> cmd/1, Selector4/1
  outer cmd/1 -> Multiport Switch/4
  Bus Selector/2 -> Multiport Switch/3  "<autopilot_cmd>"
  Bus Selector/1 -> Multiport Switch/1  "<pos>"
  NEh_current/1 -> Mux1/1
  Ground/1 -> Mux1/2
  Mux1/1 -> Selector2/1
  Selector2/1 -> Multiport Switch/2
  Selector4/1 -> Demux3/1
  Demux3/1 -> NEh_cmd/1
  Demux3/2 -> cam_cmd/1
  signal_bus/1 -> Bus Selector/1

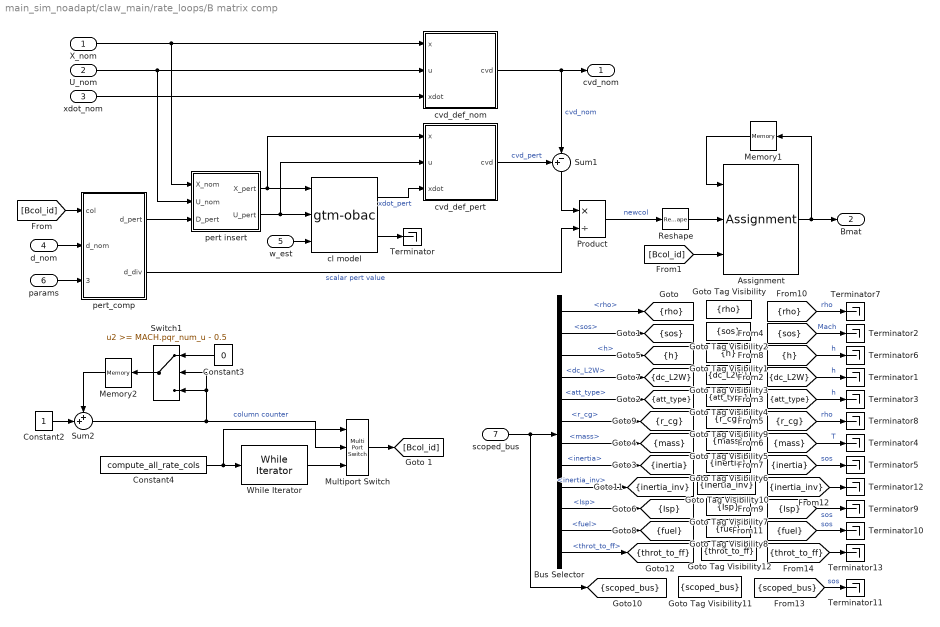
== system main_sim_noadapt/claw_main/rate_loops/B matrix comp ==
  X_nom : Inport  OutDataType=sfix(16)  OutScaling=2^0
  U_nom : Inport  Port=2  OutDataType=sfix(16)  OutScaling=2^0
  xdot_nom : Inport  Port=3  OutDataType=sfix(16)  OutScaling=2^0
  d_nom : Inport  Port=4  OutDataType=sfix(16)  OutScaling=2^0
  w_est : Inport  Port=5  OutDataType=sfix(16)  OutScaling=2^0
  params : Inport  Port=6  OutDataType=sfix(16)  OutScaling=2^0
  scoped_bus : Inport  Port=7  OutDataType=sfix(16)  OutScaling=2^0
  Assignment : Assignment  NumberOfDimensions=2  IndexOptions=Assign all,Index vector (port)  Indices=-1,1  OutputSizes=1,1
  Bus Selector : BusSelector  OutputSignals=atmos_env.rho,atmos_env.sos,atmos_env.h,dc_L2W,att_type,mass_props.r_cg,mass_props.mass,mass_props.inertia,mass_props.inertia_inv,mass_props.Isp,mass_props.fuel,mass_props.throt_to_ff
  Constant2 : Constant  OutDataType=sfix(16)  OutScaling=2^0
  Constant3 : Constant  Orientation=left  Value=0  OutDataType=sfix(16)  OutScaling=2^0
  Constant4 : Constant  Value=compute_all_rate_cols  OutDataType=sfix(16)  OutScaling=2^0
  Goto Tag Visibility : GotoTagVisibility  GotoTag=rho
  Goto Tag Visibility1 : GotoTagVisibility  GotoTag=h
  Goto Tag Visibility10 : GotoTagVisibility  GotoTag=inertia_inv
  Goto Tag Visibility11 : GotoTagVisibility  GotoTag=scoped_bus
  Goto Tag Visibility12 : GotoTagVisibility  GotoTag=throt_to_ff
  Goto Tag Visibility2 : GotoTagVisibility  GotoTag=sos
  Goto Tag Visibility3 : GotoTagVisibility  GotoTag=dc_L2W
  Goto Tag Visibility4 : GotoTagVisibility  GotoTag=att_type
  Goto Tag Visibility5 : GotoTagVisibility  GotoTag=mass
  Goto Tag Visibility6 : GotoTagVisibility  GotoTag=inertia
  Goto Tag Visibility7 : GotoTagVisibility  GotoTag=Isp
  Goto Tag Visibility8 : GotoTagVisibility  GotoTag=fuel
  Goto Tag Visibility9 : GotoTagVisibility  GotoTag=r_cg
  Memory1 : Memory  Orientation=left  X0=MACH_pqr_Bmat_IC  InheritSampleTime=on
  Memory2 : Memory  Orientation=left  InheritSampleTime=on
  Multiport Switch : MultiPortSwitch  Inputs=2  zeroidx=on
  Product : Product  Inputs=*/  OutDataType=sfix(16)  OutScaling=2^0  SaturateOnIntegerOverflow=on  InputSameDT=on  OutDataTypeStr=Inherit: Same as first input
  Reshape : Reshape  OutputDimensionality=Column vector (2-D)
  Sum1 : Sum  Orientation=down  Inputs=+-|  OutDataType=sfix(16)  OutScaling=2^0  SaturateOnIntegerOverflow=on  InputSameDT=on  OutDataTypeStr=Inherit: Same as first input
  Sum2 : Sum  Inputs=++|  OutDataType=sfix(16)  OutScaling=2^0  SaturateOnIntegerOverflow=on  InputSameDT=on  OutDataTypeStr=Inherit: Same as first input
  Switch1 : Switch  Orientation=left  Threshold=MACH.pqr_num_u - 0.5  SaturateOnIntegerOverflow=on  InputSameDT=on
  Terminator{,1..13} (14 alike) : Terminator
  While Iterator : WhileIterator  MaxIters=MACH.pqr_num_u  WhileBlockType=do-while  ShowIterationPort=on
  cl model : models/gtm-obac  SystemSampleTime=-1
  cvd_def_nom : Subsystem
  cvd_def_pert : Subsystem
  pert insert : Subsystem
  pert_comp : Subsystem
  cvd_nom : Outport  OutDataType=sfix(16)  OutScaling=2^0
  Bmat : Outport  Port=2  OutDataType=sfix(16)  OutScaling=2^0
  tag scope: Isp=scoped, att_type=scoped, dc_L2W=scoped, fuel=scoped, h=scoped, inertia=scoped, inertia_inv=scoped, mass=scoped, r_cg=scoped, rho=scoped, scoped_bus=scoped, sos=scoped, throt_to_ff=scoped
  wires:
  Reshape/1 -> Assignment/2
  pert_comp/1(d_pert) -> pert insert/3(D_pert)
  pert insert/1(X_pert) -> cvd_def_pert/1(x), cl model/1
  pert insert/2(U_pert) -> cvd_def_pert/2(u), cl model/2
  pert_comp/2(d_div) -> Product/2  "scalar pert value"
  [Bcol_id] -> pert_comp/1(col)
  Assignment/1 -> Bmat/1, Memory1/1
  [Bcol_id] -> Assignment/3
  Sum1/1 -> Product/1
  Product/1 -> Reshape/1  "newcol"
  X_nom/1 -> cvd_def_nom/1(x), pert insert/1(X_nom)
  U_nom/1 -> cvd_def_nom/2(u), pert insert/2(U_nom)
  xdot_nom/1 -> cvd_def_nom/3(xdot)
  cvd_def_pert/1(cvd) -> Sum1/1  "cvd_pert"
  cvd_def_nom/1(cvd) -> Sum1/2, cvd_nom/1  "cvd_nom"
  cl model/1 -> cvd_def_pert/3(xdot)  "xdot_pert"
  w_est/1 -> cl model/3
  d_nom/1 -> pert_comp/2(d_nom)
  Memory1/1 -> Assignment/1
  cl model/2 -> Terminator/1
  params/1 -> pert_comp/3(params)
  Constant4/1 -> Multiport Switch/1, While Iterator/1
  While Iterator/1 -> Multiport Switch/3
  Constant3/1 -> Switch1/1
  Sum2/1 -> Switch1/3, Switch1/2, Multiport Switch/2  "column counter"
  Switch1/1 -> Memory2/1
  Memory2/1 -> Sum2/1
  Constant2/1 -> Sum2/2
  Multiport Switch/1 -> [Bcol_id]
  scoped_bus/1 -> Bus Selector/1, [scoped_bus]
  [rho] -> Terminator7/1  "rho"
  [sos] -> Terminator2/1  "Mach"
  [h] -> Terminator6/1  "h"
  Bus Selector/1 -> [rho]  "<rho>"
  Bus Selector/2 -> [sos]  "<sos>"
  Bus Selector/3 -> [h]  "<h>"
  [dc_L2W] -> Terminator1/1  "h"
  Bus Selector/4 -> [dc_L2W]  "<dc_L2W>"
  [att_type] -> Terminator3/1  "h"
  Bus Selector/5 -> [att_type]  "<att_type>"
  [r_cg] -> Terminator8/1  "rho"
  [mass] -> Terminator4/1  "T"
  [inertia] -> Terminator5/1  "sos"
  Bus Selector/6 -> [r_cg]  "<r_cg>"
  Bus Selector/7 -> [mass]  "<mass>"
  Bus Selector/8 -> [inertia]  "<inertia>"
  [Isp] -> Terminator9/1  "sos"
  Bus Selector/10 -> [Isp]  "<Isp>"
  [fuel] -> Terminator10/1  "sos"
  Bus Selector/11 -> [fuel]  "<fuel>"
  [inertia_inv] -> Terminator12/1
  Bus Selector/9 -> [inertia_inv]  "<inertia_inv>"
  [scoped_bus] -> Terminator11/1  "sos"
  [throt_to_ff] -> Terminator13/1
  Bus Selector/12 -> [throt_to_ff]  "<throt_to_ff>"

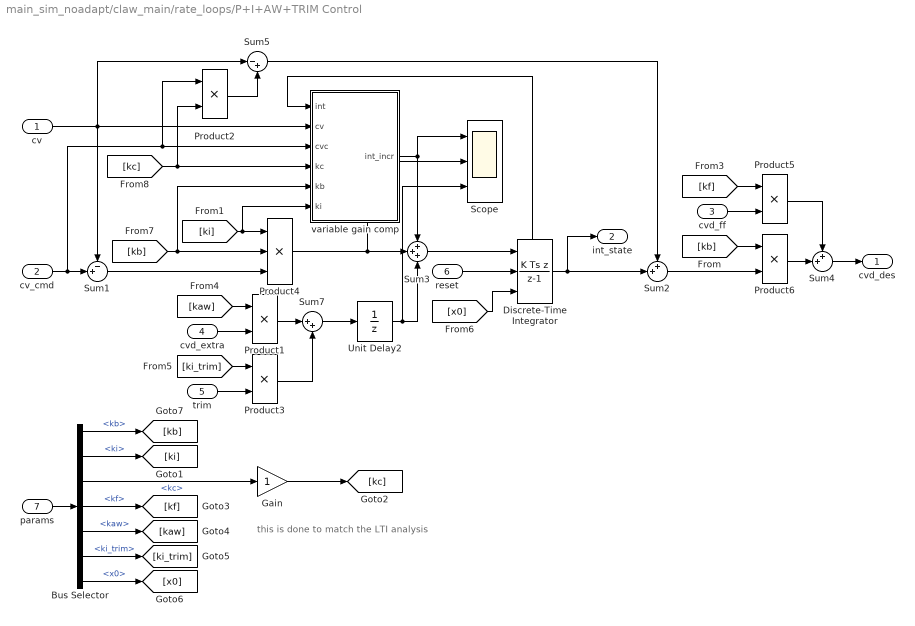
== system main_sim_noadapt/claw_main/rate_loops/P+I+AW+TRIM Control ==
  note: this is done to match the LTI analysis
  cv : Inport  OutDataType=sfix(16)  OutScaling=2^0
  cv_cmd : Inport  Port=2  OutDataType=sfix(16)  OutScaling=2^0
  cvd_ff : Inport  Port=3  OutDataType=sfix(16)  OutScaling=2^0
  cvd_extra : Inport  Port=4  OutDataType=sfix(16)  OutScaling=2^0
  trim : Inport  Port=5  OutDataType=sfix(16)  OutScaling=2^0
  reset : Inport  Port=6  OutDataType=sfix(16)  OutScaling=2^0
  params : Inport  Port=7  OutDataType=sfix(16)  OutScaling=2^0
  Bus Selector : BusSelector  OutputSignals=kb,ki,kc,kf,kaw,ki_trim,x0
  Discrete-Time Integrator : DiscreteIntegrator  IntegratorMethod=Integration: Backward Euler  ExternalReset=rising  InitialConditionSource=external  SampleTime=-1  OutDataType=sfix(16)  OutScaling=2^0  ShowStatePort=on  ICPrevOutput=DiscIntNeverNeededParam  ICPrevScaledInput=DiscIntNeverNeededParam
  Gain : Gain  ParameterDataType=sfix(16)  ParameterScaling=2^0  OutDataType=sfix(16)  OutScaling=2^0
  Product{1..3,5..6} (5 alike) : Product  OutDataType=sfix(16)  OutScaling=2^0  RndMeth=Zero
  Product4 : Product  Inputs=3  OutDataType=sfix(16)  OutScaling=2^0  RndMeth=Zero
  Scope : Scope  NumInputPorts=3
      settings: YMin=-1~-0.2~-1.25e-015  YMax=1~0.35~1.5e-015  SaveName=ScopeData27
  Sum1 : Sum  Inputs=-+|  OutDataType=sfix(16)  OutScaling=2^0  SaturateOnIntegerOverflow=on  InputSameDT=on  OutDataTypeStr=Inherit: Same as first input
  Sum2 : Sum  Inputs=++|  OutDataType=sfix(16)  OutScaling=2^0  SaturateOnIntegerOverflow=on  InputSameDT=on  OutDataTypeStr=Inherit: Same as first input
  Sum3 : Sum  Inputs=+++  OutDataType=sfix(16)  OutScaling=2^0  SaturateOnIntegerOverflow=on  InputSameDT=on  OutDataTypeStr=Inherit: Same as first input
  Sum4 : Sum  Inputs=++|  OutDataType=sfix(16)  OutScaling=2^0  SaturateOnIntegerOverflow=on  InputSameDT=on  OutDataTypeStr=Inherit: Same as first input
  Sum5 : Sum  Inputs=|-+  OutDataType=sfix(16)  OutScaling=2^0  SaturateOnIntegerOverflow=on  InputSameDT=on  OutDataTypeStr=Inherit: Same as first input
  Sum7 : Sum  Inputs=|++  OutDataType=sfix(16)  OutScaling=2^0  SaturateOnIntegerOverflow=on  InputSameDT=on  OutDataTypeStr=Inherit: Same as first input
  Unit Delay2 : UnitDelay  SampleTime=-1
  variable gain comp : Subsystem
  cvd_des : Outport  OutDataType=sfix(16)  OutScaling=2^0
  int_state : Outport  Port=2  OutDataType=sfix(16)  OutScaling=2^0
  wires:
  cv_cmd/1 -> Sum1/2, Product2/1, variable gain comp/3(cvc)
  [kb] -> variable gain comp/5(kb), Product4/2
  Sum5/1 -> Sum2/1
  Product2/1 -> Sum5/2
  [kc] -> Product2/2, variable gain comp/4(kc)
  Discrete-Time Integrator/State -> variable gain comp/1(int)
  variable gain comp/1(int_incr) -> Sum3/1, Scope/1
  Product4/1 -> Sum3/2, Scope/2
  Sum2/1 -> Product6/2
  cv/1 -> variable gain comp/2(cv), Sum5/1, Sum1/1
  Bus Selector/7 -> [x0]  "<x0>"
  params/1 -> Bus Selector/1
  [kf] -> Product5/1
  cvd_ff/1 -> Product5/2
  [kb] -> Product6/1
  [ki] -> variable gain comp/6(ki), Product4/1
  Sum1/1 -> Product4/3
  [ki_trim] -> Product3/1
  Product1/1 -> Sum7/1
  [kaw] -> Product1/1
  Bus Selector/6 -> [ki_trim]  "<ki_trim>"
  Bus Selector/5 -> [kaw]  "<kaw>"
  Bus Selector/4 -> [kf]  "<kf>"
  Bus Selector/3 -> Gain/1  "<kc>"
  Bus Selector/2 -> [ki]  "<ki>"
  Bus Selector/1 -> [kb]  "<kb>"
  Sum7/1 -> Unit Delay2/1
  Product3/1 -> Sum7/2
  reset/1 -> Discrete-Time Integrator/2
  cvd_extra/1 -> Product1/2
  Discrete-Time Integrator/1 -> Sum2/2, int_state/1
  Sum3/1 -> Discrete-Time Integrator/1
  Unit Delay2/1 -> Sum3/3, Scope/3
  trim/1 -> Product3/2
  Product6/1 -> Sum4/2
  Sum4/1 -> cvd_des/1
  Product5/1 -> Sum4/1
  [x0] -> Discrete-Time Integrator/3
  Gain/1 -> [kc]

== system main_sim_noadapt/claw_main/rate_loops/allocation ==
  cvd_nom : Inport  OutDataType=sfix(16)  OutScaling=2^0
  Bmat : Inport  Port=2  OutDataType=sfix(16)  OutScaling=2^0
  d_old : Inport  Port=3  OutDataType=sfix(16)  OutScaling=2^0
  d_nom : Inport  Port=4  OutDataType=sfix(16)  OutScaling=2^0
  cvd_des : Inport  Port=5  OutDataType=sfix(16)  OutScaling=2^0
  params : Inport  Port=6  OutDataType=sfix(16)  OutScaling=2^0
  Bmat_rcs : Selector  NumberOfDimensions=2  InputPortWidth=MACH.num_u  IndexOptions=Select all,Index vector (dialog)  Indices=-1,MACH.pqr_u_rcs_idx  OutputSizes=1
  Bmat_smn : Selector  NumberOfDimensions=2  InputPortWidth=MACH.num_u  IndexOptions=Select all,Index vector (dialog)  Indices=-1,MACH.pqr_u_smn_idx  OutputSizes=1
  Gain : Gain  Gain=-1  ParameterDataType=sfix(16)  ParameterScaling=2^0  OutDataType=sfix(16)  OutScaling=2^0
  Mux3 : Mux  Inputs=2
  RCS allocation : Subsystem
  Selector : Selector  NumberOfDimensions=2  InputPortWidth=MACH.num_u  IndexOptions=Index vector (dialog),Index vector (dialog)  Indices=1:9,1:2  OutputSizes=1
  config_di : Subsystem  BlockChoice=di_smn  mask{num_cv=MACH.pqr_num_cv, num_u=MACH.pqr_num_u_smn, wght_cv_type=MACH.pqr_wght_cv_type}
      link override di_smn/config_smn/smn_sfunc: sfunc_name=MACH.smn_sfunc_name
      settings: AttributesFormatString=%<BlockChoice>  TemplateBlock=mach_lib/config_di  MemberBlocks=di_pseudoinv,di_smn
  d_nom_smn : Selector  InputPortWidth=MACH.pqr_num_u  IndexOptions=Index vector (dialog)  Indices=MACH.pqr_u_smn_idx  OutputSizes=1
  d_old_rcs : Selector  InputPortWidth=MACH.pqr_num_u  IndexOptions=Index vector (dialog)  Indices=MACH.pqr_u_rcs_idx  OutputSizes=1
  d_old_smn : Selector  InputPortWidth=MACH.pqr_num_u  IndexOptions=Index vector (dialog)  Indices=MACH.pqr_u_smn_idx  OutputSizes=1
  param select rcs : Subsystem  mask{idx=MACH.pqr_u_rcs_idx}
      mask prompts: idx "index"
  param select smn : Subsystem  mask{idx=MACH.pqr_u_smn_idx}
      mask prompts: idx "index"
  d_cmd : Outport  OutDataType=sfix(16)  OutScaling=2^0
  cvd_extra_smn : Outport  Port=2  OutDataType=sfix(16)  OutScaling=2^0
  lambda : Outport  Port=3  OutDataType=sfix(16)  OutScaling=2^0
  solve_dat : Outport  Port=4  OutDataType=sfix(16)  OutScaling=2^0
  cvd_extra : Outport  Port=5  OutDataType=sfix(16)  OutScaling=2^0
  wires:
  config_di/1(d_cmd) -> Mux3/1
  d_nom_smn/1 -> config_di/4(d_nom)
  d_old_smn/1 -> config_di/3(d_old)
  Bmat_rcs/1 -> RCS allocation/1(Bmat)
  [Bmat] -> Bmat_rcs/1
  RCS allocation/1(rcs_cmd) -> Mux3/2
  d_old_rcs/1 -> RCS allocation/2(rcs_cmd_old)
  Bmat_smn/1 -> config_di/2(Bmat)
  Gain/1 -> RCS allocation/3(cvd_des)
  [d_old] -> d_old_rcs/1
  config_di/2(cvd_extra) -> Gain/1, cvd_extra_smn/1  "cvdex_smn"
  config_di/4(solve_dat) -> Selector/1
  cvd_nom/1 -> config_di/1(cvd_nom)
  Bmat/1 -> Bmat_smn/1, [Bmat]
  d_nom/1 -> d_nom_smn/1
  Mux3/1 -> d_cmd/1
  d_old/1 -> d_old_smn/1, [d_old]
  config_di/3(lambda) -> lambda/1
  cvd_des/1 -> config_di/5(cvd_des)
  RCS allocation/2(cvd_extra) -> cvd_extra/1
  param select smn/1(params) -> config_di/6(params)
  Selector/1 -> solve_dat/1
  params/1 -> param select smn/1(params_all), param select rcs/1(params_all)
  param select rcs/1(params) -> RCS allocation/4(params)

== system main_sim_noadapt/claw_main/rate_loops/bangbang ==
  enable_bb : Inport  OutDataType=sfix(16)  OutScaling=2^0
  att_cvc : Inport  Port=2  OutDataType=sfix(16)  OutScaling=2^0
  att_cv : Inport  Port=3  OutDataType=sfix(16)  OutScaling=2^0
  pqr : Inport  Port=4  OutDataType=sfix(16)  OutScaling=2^0
  cvd_des_lin : Inport  Port=5  OutDataType=sfix(16)  OutScaling=2^0
  Bang Bang : Stateflow chart
  Constant1 : Constant  Value=bb_params  OutDataType=sfix(16)  OutScaling=2^0
  Constant2 : Constant  Value=bb_ellipsoid  OutDataType=sfix(16)  OutScaling=2^0
  Mux : Mux  Inputs=[12 3 3 1 1 3]
  Unit Delay : UnitDelay  X0=[ 0 0 0 ]  SampleTime=MACH.dt
  Unit Delay1 : UnitDelay  SampleTime=MACH.dt
  Unit Delay2 : UnitDelay  SampleTime=MACH.dt
  cvd_des : Outport  OutDataType=sfix(16)  OutScaling=2^0
  bb_debug : Outport  Port=2  OutDataType=sfix(16)  OutScaling=2^0
  wires:
  att_cvc/1 -> Bang Bang/3(att_cvc)
  pqr/1 -> Bang Bang/5(pqr)
  att_cv/1 -> Bang Bang/4(att_cv)
  Unit Delay1/1 -> Bang Bang/11(timer_old)
  Bang Bang/5(timer) -> Unit Delay1/1, Mux/5
  Bang Bang/3(dir) -> Unit Delay/1, Mux/3
  Unit Delay/1 -> Bang Bang/9(dir_old)
  Constant1/1 -> Bang Bang/1(bb_params)
  [inertia] -> Bang Bang/6(inertia)
  enable_bb/1 -> Bang Bang/7(enable_bb)
  Unit Delay2/1 -> Bang Bang/10(use_bb_old)
  Bang Bang/4(use_bb) -> Unit Delay2/1, Mux/4
  cvd_des_lin/1 -> Bang Bang/8(cvddes_lin), Mux/6  "cvd_des_lin"
  Constant2/1 -> Bang Bang/2(bb_ellipsoid)
  Bang Bang/1(debug_output) -> Mux/1
  Mux/1 -> bb_debug/1
  Bang Bang/2(cvddes) -> cvd_des/1, Mux/2  "cvd_des"

== system main_sim_noadapt/claw_main/rate_loops/compute trim ==
  inner cmd : Inport  OutDataType=sfix(16)  OutScaling=2^0
  Bmat : Inport  Port=2  OutDataType=sfix(16)  OutScaling=2^0
  cmd : Inport  Port=3  OutDataType=sfix(16)  OutScaling=2^0
  Product : Product  Multiplication=Matrix(*)  OutDataType=sfix(16)  OutScaling=2^0  SaturateOnIntegerOverflow=on  OutDataTypeStr=Inherit: Same as first input
  Sum1 : Sum  Inputs=|+-  OutDataType=sfix(16)  OutScaling=2^0  SaturateOnIntegerOverflow=on
  trim : Outport  OutDataType=sfix(16)  OutScaling=2^0
  wires:
  Product/1 -> trim/1
  Bmat/1 -> Product/1
  Sum1/1 -> Product/2
  inner cmd/1 -> Sum1/1
  cmd/1 -> Sum1/2

== system main_sim_noadapt/claw_main/rate_loops/select rate cmd ==
  pqr_current : Inport  OutDataType=sfix(16)  OutScaling=2^0
  throt_current : Inport  Port=2  OutDataType=sfix(16)  OutScaling=2^0
  outer cmd : Inport  Port=3  OutDataType=sfix(16)  OutScaling=2^0
  signal_bus : Inport  Port=4  OutDataType=sfix(16)  OutScaling=2^0
  Bus Selector6 : BusSelector  OutputSignals=cmd_bus.select_cmd.rate
  Demux : Demux  Outputs=[ MACH.pqr_num_cv MACH.num_u_throt ]
  Multiport Switch : MultiPortSwitch  zeroidx=on  SaturateOnIntegerOverflow=on
  Mux1 : Mux  Inputs=2
  Unit Delay1 : UnitDelay  X0=MACH_throttle_IC  SampleTime=-1
  get direct cmd : Subsystem
  select multiple throts : Selector  InputPortWidth=4  IndexOptions=Index vector (dialog)  Indices=[1:3 4*ones(1,MACH.num_u_throt)]  OutputSizes=1
  pqr_cmd : Outport  OutDataType=sfix(16)  OutScaling=2^0
  throt_cmd : Outport  Port=2  OutDataType=sfix(16)  OutScaling=2^0
  cmd : Outport  Port=3  OutDataType=sfix(16)  OutScaling=2^0
  wires:
  Multiport Switch/1 -> cmd/1, Demux/1
  outer cmd/1 -> Multiport Switch/4
  Mux1/1 -> Multiport Switch/2
  select multiple throts/1 -> Multiport Switch/1
  Unit Delay1/1 -> Mux1/2
  pqr_current/1 -> Mux1/1
  throt_current/1 -> Unit Delay1/1
  get direct cmd/1(direct_cmd) -> Multiport Switch/3
  signal_bus/1 -> get direct cmd/1(signal_bus), Bus Selector6/1
  Bus Selector6/1 -> select multiple throts/1  "<rate>"
  Demux/1 -> pqr_cmd/1
  Demux/2 -> throt_cmd/1

== system main_sim_noadapt/claw_main/rate_loops/set rate loop params ==
  rate_params : Inport  OutDataType=sfix(16)  OutScaling=2^0
  u_old : Inport  Port=2  OutDataType=sfix(16)  OutScaling=2^0
  Bus Assignment : BusAssignment  AssignedSignals=u_ulim,u_llim
  Bus Selector1 : BusSelector  OutputSignals=u_ulim,u_llim,u_urlim,u_lrlim
  rate limit limits : mach_lib/rate limit limits  SystemSampleTime=-1  ulim=MACH.pqr_u_ulim  llim=MACH.pqr_u_llim
  params : Outport  OutDataType=sfix(16)  OutScaling=2^0
  wires:
  u_old/1 -> rate limit limits/1
  rate_params/1 -> Bus Selector1/1, Bus Assignment/1
  Bus Selector1/1 -> rate limit limits/2  "<u_ulim>"
  Bus Selector1/2 -> rate limit limits/3  "<u_llim>"
  Bus Selector1/3 -> rate limit limits/4  "<u_urlim>"
  Bus Selector1/4 -> rate limit limits/5  "<u_lrlim>"
  rate limit limits/1 -> Bus Assignment/2
  rate limit limits/2 -> Bus Assignment/3
  Bus Assignment/1 -> params/1

== system main_sim_noadapt/claw_main/servo commands  when not engaged/pseudo surf cmd ==
  autopilot_cmd : Inport  OutDataType=sfix(16)  OutScaling=2^0
  Assignment1 : Assignment  IndexOptions=Index vector (dialog)  Indices=[ MACH.vane_idx MACH.throttle_idx ]  OutputSizes=[1 1]
  Constant : Constant  Value=MACH_U_nom_IC  OutDataType=sfix(16)  OutScaling=2^0
  Demux2 : Demux  Outputs=[ 3 1 ]
  Gain : Gain  Gain=MACH.mixer  Multiplication=Matrix(K*u)  ParameterDataType=sfix(16)  ParameterScaling=2^0  OutDataType=sfix(16)  OutScaling=2^0  SaturateOnIntegerOverflow=on  OutDataTypeStr=Inherit: Same as input  ParamDataTypeStr=Inherit: Same as input
  Gain1 : Gain  Gain=MACH.throt_mixer  ParameterDataType=sfix(16)  ParameterScaling=2^0  OutDataType=sfix(16)  OutScaling=2^0
  Mux : Mux  Inputs=2
  surf_cmd : Outport  OutDataType=sfix(16)  OutScaling=2^0
  wires:
  Mux/1 -> Assignment1/2
  Gain1/1 -> Mux/2
  Gain/1 -> Mux/1
  Demux2/2 -> Gain1/1  "throttle"
  Demux2/1 -> Gain/1  "da,de,dr"
  autopilot_cmd/1 -> Demux2/1
  Assignment1/1 -> surf_cmd/1
  Constant/1 -> Assignment1/1
